simulink model "Counter"  (R2021a)
settings: Solver=FixedStepDiscrete  StartTime=0.0  StopTime=10  RelTol=1e-3
model workspace (MAT data in the model file):
  MAX = 10
  threshold = 0
settings Model: Creator=OmarMedhat  LastModifiedBy=OmarMedhat
settings OptimizationCC: DefaultParameterBehavior=Inlined  EnhancedBackFolding=on  PassReuseOutputArgsAs=Individual arguments  ZeroExternalMemoryAtStartup=off  ZeroInternalMemoryAtStartup=off  OptimizeBlockOrder=speed  DifferentSizesBufferReuse=on  OptimizationCustomize=off  EfficientTunableParamExpr=on
settings DebuggingCC: ParameterTunabilityLossMsg=error
settings SFSimCC: MATLABDynamicMemAlloc=off
settings RTWCC: SystemTargetFile=ert.tlc  GenCodeOnly=on  TemplateMakefile=ert_default_tmf  GenerateReport=on  IncludeHyperlinkInReport=on  LaunchReport=on  GenerateTraceInfo=on
settings CodeAppCC: ForceParamTrailComments=on  IgnoreCustomStorageClasses=off  OperatorAnnotations=on  SimulinkDataObjDesc=on  SFDataObjDesc=on  InsertBlockDesc=on
settings ERTTargetCC: TargetLangStandard=C99 (ISO)  GenerateSampleERTMain=on  InlinedParameterPlacement=NonHierarchical  ERTCustomFileTemplate=example_file_process.tlc

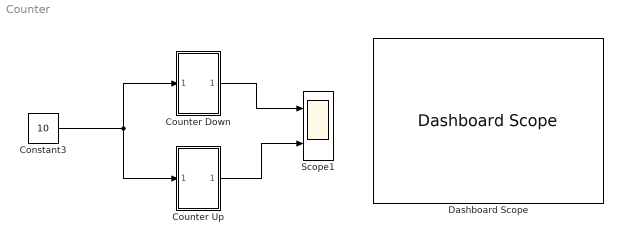
== system Counter ==
  Constant3 : Constant  Value=10
  Counter Down : Subsystem
  Counter Up : Subsystem
  Dashboard Scope : DashboardScope
  Scope1 : Scope  NumInputPorts=2
  wires:
  Constant3/1 -> Counter Up/1(In1), Counter Down/1(In1)
  Counter Up/1(Out1) -> Scope1/2
  Counter Down/1(Out1) -> Scope1/1

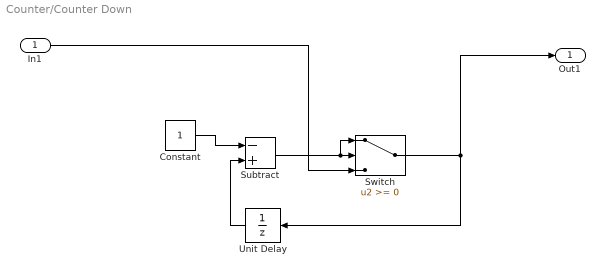
== system Counter/Counter Down ==
  In1 : Inport
  Constant : Constant
  Subtract : Sum  Inputs=-+
  Switch : Switch
  Unit Delay : UnitDelay  SampleTime=-1  HasFrameUpgradeWarning=on
  Out1 : Outport
  wires:
  Subtract/1 -> Switch/1, Switch/2
  Unit Delay/1 -> Subtract/2
  Constant/1 -> Subtract/1
  Switch/1 -> Out1/1, Unit Delay/1
  In1/1 -> Switch/3

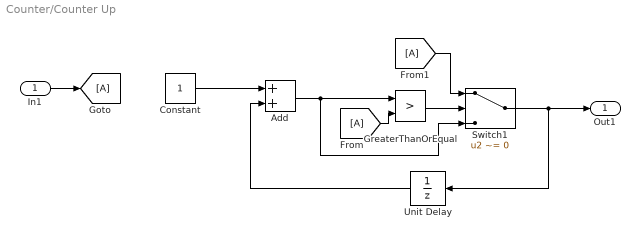
== system Counter/Counter Up ==
  In1 : Inport
  Add : Sum
  Constant : Constant
  GreaterThanOrEqual : RelationalOperator  Operator=>  OutDataTypeStr=boolean  RndMeth=Simplest
  Switch1 : Switch  Criteria=u2 ~= 0
  Unit Delay : UnitDelay  InitialCondition=-1  HasFrameUpgradeWarning=on
  Out1 : Outport
  wires:
  Add/1 -> Switch1/3, GreaterThanOrEqual/1
  In1/1 -> [A]
  Switch1/1 -> Out1/1, Unit Delay/1
  GreaterThanOrEqual/1 -> Switch1/2
  Constant/1 -> Add/1
  [A] -> GreaterThanOrEqual/2
  Unit Delay/1 -> Add/2
  [A] -> Switch1/1
